simulink model "minmax_basic"  (Simulink 6.6)
settings: Solver=FixedStepDiscrete  StartTime=0.0  StopTime=10.0  FixedStep=1  RelTol=1e-3
settings Model: Creator=Nyenyec  LastModifiedBy=hnine

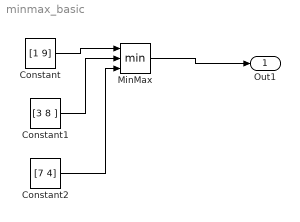
== system minmax_basic ==
  Constant : Constant  Value=[1 9]
  Constant1 : Constant  Value=[3 8 ]
  Constant2 : Constant  Value=[7 4]
  MinMax : MinMax  Inputs=3
  Out1 : Outport
  wires:
  Constant/1 -> MinMax/1
  Constant1/1 -> MinMax/2
  Constant2/1 -> MinMax/3
  MinMax/1 -> Out1/1
